simulink model "ds_capital_nonlinear_1o_simulation_simu"  (R2022b)
settings: Solver=FixedStepAuto  StartTime=0.0  StopTime=N*time_step  FixedStep=5  RelTol=1e-3
values from neighbouring files (symbols this model uses):
  A = 1    [ds_capital_nonlinear_1o_simulation_data.mat]
  B = [0.0344686419902 0.0344686419902 0.0344686419902 -0.0344686419902]    [ds_capital_nonlinear_1o_simulation_data.mat]
  C = 0.25    [ds_capital_nonlinear_1o_simulation_data.mat]
  D = [0.00832931278442 0.00357068771392 0.00406727923079 -0.697078431224]    [ds_capital_nonlinear_1o_simulation_data.mat]
  OR = [0.65 0.49 9.81 0.7 0]    [ds_capital_nonlinear_1o_simulation_data.mat]
settings Model: Creator=chuan  LastModifiedBy=chuan

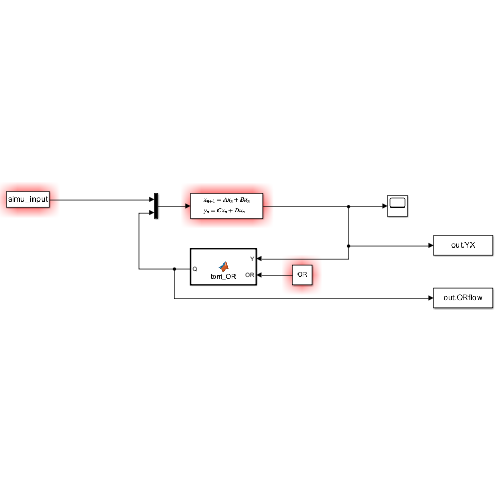
[thumbnail: Simulink's stored preview of the top-level diagram]
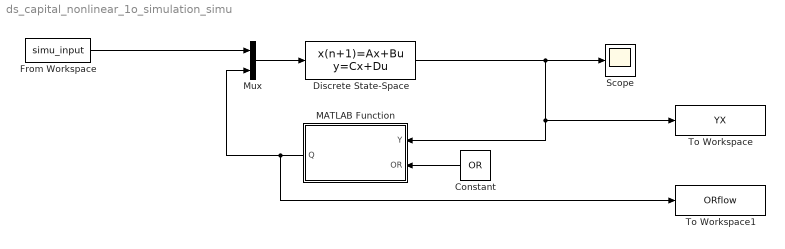
== system ds_capital_nonlinear_1o_simulation_simu ==
  Constant : Constant  Value=OR
  Discrete State-Space : DiscreteStateSpace  A=A  B=B  C=C  D=D  SampleTime=-1
  From Workspace : FromWorkspace  VariableName=simu_input  SampleTime=-1
  MATLAB Function : MATLAB Function  TreatAsAtomicUnit=on
  Mux : Mux  Inputs=2
  Scope : Scope
  To Workspace : ToWorkspace  VariableName=YX  SaveFormat=Timeseries  SampleTime=-1
  To Workspace1 : ToWorkspace  VariableName=ORflow  SaveFormat=Timeseries  SampleTime=-1
  wires:
  Discrete State-Space/1 -> MATLAB Function/1(Y), To Workspace/1, Scope/1
  Mux/1 -> Discrete State-Space/1
  Constant/1 -> MATLAB Function/2(OR)
  MATLAB Function/1(Q) -> Mux/2, To Workspace1/1
  From Workspace/1 -> Mux/1

== matlab function ds_capital_nonlinear_1o_simulation_simu/MATLAB Function ==
  data: Y input; Q output; OR input
function Q = torri_OR(Y,OR)

% Import Orifice Data
Cd = OR(1);
A0 = OR(2);
g = OR(3);
Yfull = OR(4);
Z0 = OR(5);

% Compute Outflow
constant = sqrt(32/27);
boundary = 0.25*(3*Yfull + 4*Z0);

% constant = 1;
% boundary = Yfull + Z0;

% Compute Outflow
if Y <= Z0
        Q = 0;
    elseif Y > Z0 && Y < boundary
        CwL = (Cd*A0*sqrt(g))/(Yfull);
        CwL = constant*CwL;
        Q = CwL*(Y-Z0)^(1.5);
    else
        He = Y-(Z0 + Yfull/2);
        Q = Cd*A0*sqrt(2*g*He);
end

end
